simulink subsystem "Airdata"  (R2024b)
settings: Solver=VariableStepAuto  StartTime=0.0  StopTime=10.0  RelTol=1e-3
libraries: aerolibasang x2
settings Model: Creator=joedo  LastModifiedBy=finnb

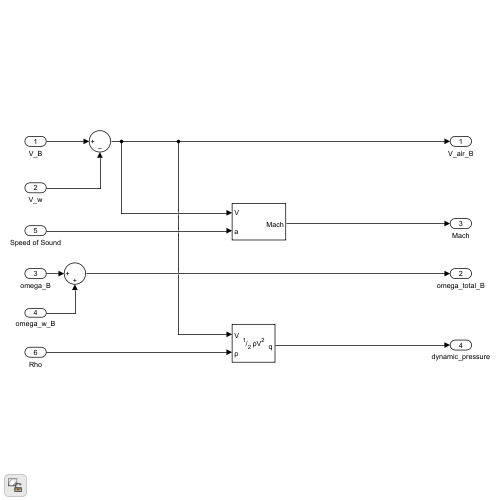
[thumbnail: Simulink's stored preview of the top-level diagram]
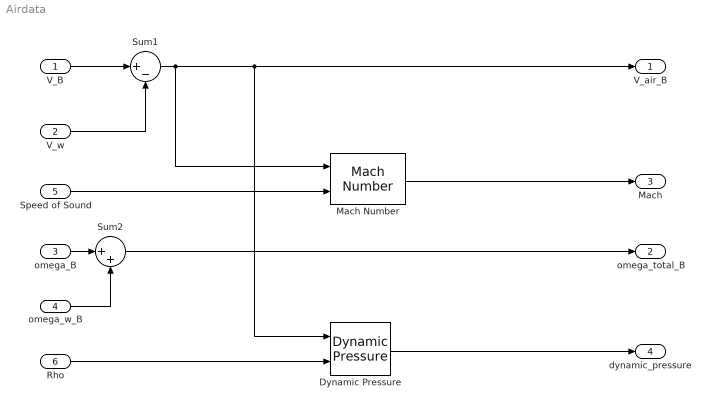
== system Airdata ==
  V_B : Inport
  V_w : Inport  Port=2
  omega_B : Inport  Port=3
  omega_w_B : Inport  Port=4
  Speed of Sound : Inport  Port=5  Unit=m/s
  Rho : Inport  Port=6  Unit=m/s
  Dynamic Pressure : aerolibasang/Dynamic Pressure
  Mach Number : aerolibasang/Mach Number
  Sum1 : Sum  Inputs=|+-  InputSameDT=on  SaturateOnIntegerOverflow=on  OutDataTypeStr=Inherit: Same as first input
  Sum2 : Sum  Inputs=|++  InputSameDT=on  SaturateOnIntegerOverflow=on  OutDataTypeStr=Inherit: Same as first input
  V_air_B : Outport  VectorParamsAs1DForOutWhenUnconnected=off
  omega_total_B : Outport  Port=2  VectorParamsAs1DForOutWhenUnconnected=off
  Mach : Outport  Port=3  VectorParamsAs1DForOutWhenUnconnected=off
  dynamic_pressure : Outport  Port=4  VectorParamsAs1DForOutWhenUnconnected=off
  wires:
  V_w/1 -> Sum1/2
  omega_B/1 -> Sum2/1
  omega_w_B/1 -> Sum2/2
  Sum2/1 -> omega_total_B/1
  V_B/1 -> Sum1/1
  Mach Number/1 -> Mach/1
  Sum1/1 -> V_air_B/1, Dynamic Pressure/1, Mach Number/1
  Speed of Sound/1 -> Mach Number/2
  Rho/1 -> Dynamic Pressure/2
  Dynamic Pressure/1 -> dynamic_pressure/1
